simulink model "humanSubject07_48dof_test"  (R2022a)
settings: Solver=VariableStepAuto  StartTime=0.0  StopTime=4.5  RelTol=1e-3
values from neighbouring files (symbols this model uses):
  m = size(marker.links, 1)    [master_thesis_script.m]    (also in trial.m)
  marker = msg.ChildFrameId(14)    [callback_class.m]
  noise =     [noise_S1_F1_H2.mat]    (also in show_Results.m = noise.noise)
  s = s + 1    (= 2)    [Phi_J_generation.m]    (also in master_thesis_script.m; trial.m)
undefined symbols (not defined in the file or in its folder): arm, LS, X, Y, Z
libraries: nesl_utility x105, sm_lib x84
(part 2 of 3)

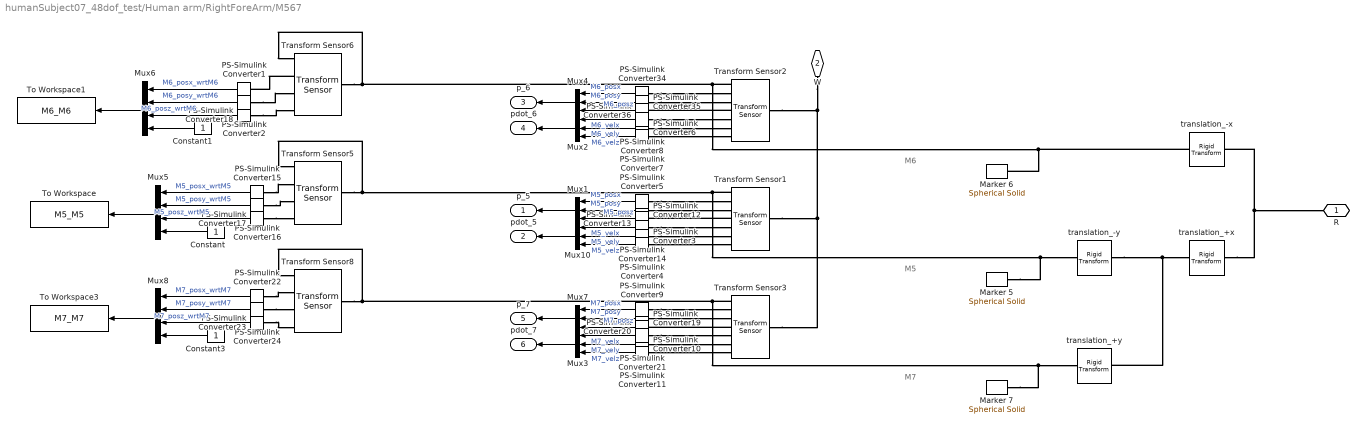
== system humanSubject07_48dof_test/Human arm/RightForeArm/M567 ==
  note: M6
  note: M5
  note: M7
  Constant : Constant
  Constant1 : Constant
  Constant3 : Constant
  Marker 5 : sm_lib/Body Elements/Spherical Solid  GraphicAmbientColor=[0.15 0.15 0.15 1.0]  BasedOnType=Density  CenterOfMass=[0 0 0]  CenterOfMassUnits=m  GraphicDiffuseColor=[1.0 0.2 0.2]  Density=1000  DensityUnits=kg/m^3  DoExposeReferenceFrame=on  GraphicEmissiveColor=[0.0 0.0 0.0 1.0]  ExportEntireGeometry=off  SerializedExposedGeometries=<ExposedGeometries/>  SerializedFrames=<Frames/>  MarkerShape=Sphere  MarkerSize=10  GraphicType=FromGeometry  InertiaType=CalculateFromGeometry  Mass=1  MassUnits=kg  MomentsOfInertia=[1 1 1]  MomentsOfInertiaUnits=kg*m^2  GraphicOpacity=1.0  ProductsOfInertia=[0 0 0]  ProductsOfInertiaUnits=kg*m^2  GraphicShininess=75  GraphicSpecularColor=[0.5 0.5 0.5 1.0]  SphereRadius=arm.markers.radius  SphereRadiusUnits=m  GraphicVisPropType=SimpleVisualProperties
  Marker 6 : sm_lib/Body Elements/Spherical Solid  GraphicAmbientColor=[0.15 0.15 0.15 1.0]  BasedOnType=Density  CenterOfMass=[0 0 0]  CenterOfMassUnits=m  GraphicDiffuseColor=[1.0 0.2 0.2]  Density=1000  DensityUnits=kg/m^3  DoExposeReferenceFrame=on  GraphicEmissiveColor=[0.0 0.0 0.0 1.0]  ExportEntireGeometry=off  SerializedExposedGeometries=<ExposedGeometries/>  SerializedFrames=<Frames/>  MarkerShape=Sphere  MarkerSize=10  GraphicType=FromGeometry  InertiaType=CalculateFromGeometry  Mass=1  MassUnits=kg  MomentsOfInertia=[1 1 1]  MomentsOfInertiaUnits=kg*m^2  GraphicOpacity=1.0  ProductsOfInertia=[0 0 0]  ProductsOfInertiaUnits=kg*m^2  GraphicShininess=75  GraphicSpecularColor=[0.5 0.5 0.5 1.0]  SphereRadius=arm.markers.radius  SphereRadiusUnits=m  GraphicVisPropType=SimpleVisualProperties
  Marker 7 : sm_lib/Body Elements/Spherical Solid  GraphicAmbientColor=[0.15 0.15 0.15 1.0]  BasedOnType=Density  CenterOfMass=[0 0 0]  CenterOfMassUnits=m  GraphicDiffuseColor=[1.0 0.2 0.2]  Density=1000  DensityUnits=kg/m^3  DoExposeReferenceFrame=on  GraphicEmissiveColor=[0.0 0.0 0.0 1.0]  ExportEntireGeometry=off  SerializedExposedGeometries=<ExposedGeometries/>  SerializedFrames=<Frames/>  MarkerShape=Sphere  MarkerSize=10  GraphicType=FromGeometry  InertiaType=CalculateFromGeometry  Mass=1  MassUnits=kg  MomentsOfInertia=[1 1 1]  MomentsOfInertiaUnits=kg*m^2  GraphicOpacity=1.0  ProductsOfInertia=[0 0 0]  ProductsOfInertiaUnits=kg*m^2  GraphicShininess=75  GraphicSpecularColor=[0.5 0.5 0.5 1.0]  SphereRadius=arm.markers.radius  SphereRadiusUnits=m  GraphicVisPropType=SimpleVisualProperties
  Mux{1..4,7,10} (6 alike) : Mux  Inputs=3
  Mux5 : Mux
  Mux6 : Mux
  Mux8 : Mux
  PS-Simulink Converter{1..24,34..36} (27 alike) : nesl_utility/PS-Simulink Converter  PhysicalDomain=network_engine_domain  SubClassName=ps_output  LeftPortType=input  RightPortType=output  PseudoPeriodic=off  Frequencies=[]  VectorFormat=inherit  Unit=inherit  AffineConversion=off
      settings: SourceProductBaseCode=SS,PW,VE
  To Workspace : ToWorkspace  VariableName=M5_M5  SaveFormat=Structure With Time  SampleTime=-1
  To Workspace1 : ToWorkspace  VariableName=M6_M6  SaveFormat=Structure With Time  SampleTime=-1
  To Workspace3 : ToWorkspace  VariableName=M7_M7  SaveFormat=Structure With Time  SampleTime=-1
  Transform Sensor1 : sm_lib/Frames and Transforms/Transform Sensor  MeasurementFrame=World  SenseAngle=off  SenseAxis=off  SenseAngle1=off  SenseAngle2=off  SenseAngle3=off  SenseQ=off  SenseR=off  SenseOmegaX=off  SenseOmegaY=off  SenseOmegaZ=off  SenseOmega1=off  SenseOmega2=off  SenseOmega3=off  SenseQDot=off  SenseRDot=off  SenseAlphaX=off  SenseAlphaY=off  SenseAlphaZ=off  SenseAlpha1=off  SenseAlpha2=off  SenseAlpha3=off  SenseQDDot=off  SenseRDDot=off  SenseX=on  SenseY=on  SenseZ=on  SenseRad=off  SenseAzim=off  SenseDist=off  SenseInc=off  SenseXDot=on  SenseYDot=on  SenseZDot=on  SenseRadDot=off  SenseAzimDot=off  SenseDistDot=off  SenseIncDot=off  SenseXDDot=off  SenseYDDot=off  SenseZDDot=off  SenseRadDDot=off  SenseAzimDDot=off  SenseDistDDot=off  SenseIncDDot=off
  Transform Sensor2 : sm_lib/Frames and Transforms/Transform Sensor  MeasurementFrame=World  SenseAngle=off  SenseAxis=off  SenseAngle1=off  SenseAngle2=off  SenseAngle3=off  SenseQ=off  SenseR=off  SenseOmegaX=off  SenseOmegaY=off  SenseOmegaZ=off  SenseOmega1=off  SenseOmega2=off  SenseOmega3=off  SenseQDot=off  SenseRDot=off  SenseAlphaX=off  SenseAlphaY=off  SenseAlphaZ=off  SenseAlpha1=off  SenseAlpha2=off  SenseAlpha3=off  SenseQDDot=off  SenseRDDot=off  SenseX=on  SenseY=on  SenseZ=on  SenseRad=off  SenseAzim=off  SenseDist=off  SenseInc=off  SenseXDot=on  SenseYDot=on  SenseZDot=on  SenseRadDot=off  SenseAzimDot=off  SenseDistDot=off  SenseIncDot=off  SenseXDDot=off  SenseYDDot=off  SenseZDDot=off  SenseRadDDot=off  SenseAzimDDot=off  SenseDistDDot=off  SenseIncDDot=off
  Transform Sensor3 : sm_lib/Frames and Transforms/Transform Sensor  MeasurementFrame=World  SenseAngle=off  SenseAxis=off  SenseAngle1=off  SenseAngle2=off  SenseAngle3=off  SenseQ=off  SenseR=off  SenseOmegaX=off  SenseOmegaY=off  SenseOmegaZ=off  SenseOmega1=off  SenseOmega2=off  SenseOmega3=off  SenseQDot=off  SenseRDot=off  SenseAlphaX=off  SenseAlphaY=off  SenseAlphaZ=off  SenseAlpha1=off  SenseAlpha2=off  SenseAlpha3=off  SenseQDDot=off  SenseRDDot=off  SenseX=on  SenseY=on  SenseZ=on  SenseRad=off  SenseAzim=off  SenseDist=off  SenseInc=off  SenseXDot=on  SenseYDot=on  SenseZDot=on  SenseRadDot=off  SenseAzimDot=off  SenseDistDot=off  SenseIncDot=off  SenseXDDot=off  SenseYDDot=off  SenseZDDot=off  SenseRadDDot=off  SenseAzimDDot=off  SenseDistDDot=off  SenseIncDDot=off
  Transform Sensor5 : sm_lib/Frames and Transforms/Transform Sensor  MeasurementFrame=World  SenseAngle=off  SenseAxis=off  SenseAngle1=off  SenseAngle2=off  SenseAngle3=off  SenseQ=off  SenseR=off  SenseOmegaX=off  SenseOmegaY=off  SenseOmegaZ=off  SenseOmega1=off  SenseOmega2=off  SenseOmega3=off  SenseQDot=off  SenseRDot=off  SenseAlphaX=off  SenseAlphaY=off  SenseAlphaZ=off  SenseAlpha1=off  SenseAlpha2=off  SenseAlpha3=off  SenseQDDot=off  SenseRDDot=off  SenseX=on  SenseY=on  SenseZ=on  SenseRad=off  SenseAzim=off  SenseDist=off  SenseInc=off  SenseXDot=off  SenseYDot=off  SenseZDot=off  SenseRadDot=off  SenseAzimDot=off  SenseDistDot=off  SenseIncDot=off  SenseXDDot=off  SenseYDDot=off  SenseZDDot=off  SenseRadDDot=off  SenseAzimDDot=off  SenseDistDDot=off  SenseIncDDot=off
  Transform Sensor6 : sm_lib/Frames and Transforms/Transform Sensor  MeasurementFrame=World  SenseAngle=off  SenseAxis=off  SenseAngle1=off  SenseAngle2=off  SenseAngle3=off  SenseQ=off  SenseR=off  SenseOmegaX=off  SenseOmegaY=off  SenseOmegaZ=off  SenseOmega1=off  SenseOmega2=off  SenseOmega3=off  SenseQDot=off  SenseRDot=off  SenseAlphaX=off  SenseAlphaY=off  SenseAlphaZ=off  SenseAlpha1=off  SenseAlpha2=off  SenseAlpha3=off  SenseQDDot=off  SenseRDDot=off  SenseX=on  SenseY=on  SenseZ=on  SenseRad=off  SenseAzim=off  SenseDist=off  SenseInc=off  SenseXDot=off  SenseYDot=off  SenseZDot=off  SenseRadDot=off  SenseAzimDot=off  SenseDistDot=off  SenseIncDot=off  SenseXDDot=off  SenseYDDot=off  SenseZDDot=off  SenseRadDDot=off  SenseAzimDDot=off  SenseDistDDot=off  SenseIncDDot=off
  Transform Sensor8 : sm_lib/Frames and Transforms/Transform Sensor  MeasurementFrame=World  SenseAngle=off  SenseAxis=off  SenseAngle1=off  SenseAngle2=off  SenseAngle3=off  SenseQ=off  SenseR=off  SenseOmegaX=off  SenseOmegaY=off  SenseOmegaZ=off  SenseOmega1=off  SenseOmega2=off  SenseOmega3=off  SenseQDot=off  SenseRDot=off  SenseAlphaX=off  SenseAlphaY=off  SenseAlphaZ=off  SenseAlpha1=off  SenseAlpha2=off  SenseAlpha3=off  SenseQDDot=off  SenseRDDot=off  SenseX=on  SenseY=on  SenseZ=on  SenseRad=off  SenseAzim=off  SenseDist=off  SenseInc=off  SenseXDot=off  SenseYDot=off  SenseZDot=off  SenseRadDot=off  SenseAzimDot=off  SenseDistDot=off  SenseIncDot=off  SenseXDDot=off  SenseYDDot=off  SenseZDDot=off  SenseRadDDot=off  SenseAzimDDot=off  SenseDistDDot=off  SenseIncDDot=off
  translation_+x : sm_lib/Frames and Transforms/Rigid Transform  TranslationMethod=Cartesian  TranslationStandardOffset=0  TranslationLengthUnit=m  TranslationStandardAxis=+Z  TranslationCartesianOffset=[arm.forearm.radius+arm.markers.radius 0 0]  TranslationROffset=0  TranslationROffsetUnits=m  TranslationZOffset=0  TranslationZOffsetUnits=m  TranslationThetaOffset=0  TranslationThetaOffsetUnits=deg  RotationMethod=None  RotationAngleUnits=rad  RotationStandardAxis=+Z  RotationAngle=pi/2  RotationArbitraryAxis=[1 0 0]  FollAlignAxisA=+X  BaseAlignAxisA=+Y  FollAlignAxisB=+Y  BaseAlignAxisB=+Z  RotationSequenceAxes=BaseAxes  RotationSequence=XYZ  RotationSequenceAngles=[pi/2, 0, 0]  RotationSequenceAnglesUnits=rad  RotationMatrix=[1 0 0; 0 1 0; 0 0 1]
  translation_+y : sm_lib/Frames and Transforms/Rigid Transform  TranslationMethod=Cartesian  TranslationStandardOffset=0  TranslationLengthUnit=m  TranslationStandardAxis=+Z  TranslationCartesianOffset=[0 arm.forearm.length/4 0]  TranslationROffset=0  TranslationROffsetUnits=m  TranslationZOffset=0  TranslationZOffsetUnits=m  TranslationThetaOffset=0  TranslationThetaOffsetUnits=deg  RotationMethod=None  RotationAngleUnits=rad  RotationStandardAxis=+Z  RotationAngle=pi/2  RotationArbitraryAxis=[1 0 0]  FollAlignAxisA=+X  BaseAlignAxisA=+Y  FollAlignAxisB=+Y  BaseAlignAxisB=+Z  RotationSequenceAxes=BaseAxes  RotationSequence=XYZ  RotationSequenceAngles=[pi/2, 0, 0]  RotationSequenceAnglesUnits=rad  RotationMatrix=[1 0 0; 0 1 0; 0 0 1]
  translation_-x : sm_lib/Frames and Transforms/Rigid Transform  TranslationMethod=Cartesian  TranslationStandardOffset=0  TranslationLengthUnit=m  TranslationStandardAxis=+Z  TranslationCartesianOffset=[-arm.forearm.radius-arm.markers.radius 0 0]  TranslationROffset=0  TranslationROffsetUnits=m  TranslationZOffset=0  TranslationZOffsetUnits=m  TranslationThetaOffset=0  TranslationThetaOffsetUnits=deg  RotationMethod=None  RotationAngleUnits=rad  RotationStandardAxis=+Z  RotationAngle=pi/2  RotationArbitraryAxis=[1 0 0]  FollAlignAxisA=+X  BaseAlignAxisA=+Y  FollAlignAxisB=+Y  BaseAlignAxisB=+Z  RotationSequenceAxes=BaseAxes  RotationSequence=XYZ  RotationSequenceAngles=[pi/2, 0, 0]  RotationSequenceAnglesUnits=rad  RotationMatrix=[1 0 0; 0 1 0; 0 0 1]
  translation_-y : sm_lib/Frames and Transforms/Rigid Transform  TranslationMethod=Cartesian  TranslationStandardOffset=0  TranslationLengthUnit=m  TranslationStandardAxis=+Z  TranslationCartesianOffset=[0 -arm.forearm.length/4 0]  TranslationROffset=0  TranslationROffsetUnits=m  TranslationZOffset=0  TranslationZOffsetUnits=m  TranslationThetaOffset=0  TranslationThetaOffsetUnits=deg  RotationMethod=None  RotationAngleUnits=rad  RotationStandardAxis=+Z  RotationAngle=pi/2  RotationArbitraryAxis=[1 0 0]  FollAlignAxisA=+X  BaseAlignAxisA=+Y  FollAlignAxisB=+Y  BaseAlignAxisB=+Z  RotationSequenceAxes=BaseAxes  RotationSequence=XYZ  RotationSequenceAngles=[pi/2, 0, 0]  RotationSequenceAnglesUnits=rad  RotationMatrix=[1 0 0; 0 1 0; 0 0 1]
  R : PMIOPort  Side=Left
  W : PMIOPort  Port=2  Side=Left
  p_5 : Outport
  pdot_5 : Outport  Port=2
  p_6 : Outport  Port=3
  pdot_6 : Outport  Port=4
  p_7 : Outport  Port=5
  pdot_7 : Outport  Port=6
  wires:
  Mux5/1 -> To Workspace/1
  PS-Simulink Converter17/1 -> Mux5/3  "M5_posz_wrtM5"
  PS-Simulink Converter15/1 -> Mux5/1  "M5_posx_wrtM5"
  PS-Simulink Converter16/1 -> Mux5/2  "M5_posy_wrtM5"
  Constant/1 -> Mux5/4
  Mux6/1 -> To Workspace1/1
  PS-Simulink Converter1/1 -> Mux6/1  "M6_posx_wrtM6"
  PS-Simulink Converter2/1 -> Mux6/2  "M6_posy_wrtM6"
  Constant1/1 -> Mux6/4
  PS-Simulink Converter18/1 -> Mux6/3  "M6_posz_wrtM6"
  Constant3/1 -> Mux8/4
  PS-Simulink Converter22/1 -> Mux8/1  "M7_posx_wrtM7"
  PS-Simulink Converter24/1 -> Mux8/2  "M7_posy_wrtM7"
  Mux8/1 -> To Workspace3/1
  PS-Simulink Converter23/1 -> Mux8/3  "M7_posz_wrtM7"
  PS-Simulink Converter35/1 -> Mux4/2  "M6_posy"
  PS-Simulink Converter34/1 -> Mux4/1  "M6_posx"
  PS-Simulink Converter8/1 -> Mux2/1  "M6_velx"
  PS-Simulink Converter6/1 -> Mux2/2  "M6_vely"
  PS-Simulink Converter36/1 -> Mux4/3  "M6_posz"
  PS-Simulink Converter7/1 -> Mux2/3  "M6_velz"
  PS-Simulink Converter12/1 -> Mux1/2  "M5_posy"
  PS-Simulink Converter5/1 -> Mux1/1  "M5_posx"
  PS-Simulink Converter14/1 -> Mux10/1  "M5_velx"
  PS-Simulink Converter3/1 -> Mux10/2  "M5_vely"
  PS-Simulink Converter13/1 -> Mux1/3  "M5_posz"
  PS-Simulink Converter4/1 -> Mux10/3  "M5_velz"
  PS-Simulink Converter19/1 -> Mux7/2  "M7_posy"
  PS-Simulink Converter9/1 -> Mux7/1  "M7_posx"
  PS-Simulink Converter21/1 -> Mux3/1  "M7_velx"
  PS-Simulink Converter10/1 -> Mux3/2  "M7_vely"
  PS-Simulink Converter20/1 -> Mux7/3  "M7_posz"
  PS-Simulink Converter11/1 -> Mux3/3  "M7_velz"
  Mux1/1 -> p_5/1
  Mux10/1 -> pdot_5/1
  Mux4/1 -> p_6/1
  Mux2/1 -> pdot_6/1
  Mux7/1 -> p_7/1
  Mux3/1 -> pdot_7/1
  connections:
  translation_+x/LConn1 -- translation_-x/LConn1 -- R/RConn1
  translation_-y/LConn1 -- translation_+y/LConn1 -- translation_+x/RConn1
  Transform Sensor2/RConn1 -- Transform Sensor6/RConn1 -- Transform Sensor6/LConn1 -- Marker 6/RConn1 -- translation_-x/RConn1
  W/RConn1 -- Transform Sensor3/LConn1 -- Transform Sensor1/LConn1 -- Transform Sensor2/LConn1
  PS-Simulink Converter16/LConn1 -- Transform Sensor5/RConn3
  PS-Simulink Converter17/LConn1 -- Transform Sensor5/RConn4
  PS-Simulink Converter15/LConn1 -- Transform Sensor5/RConn2
  Transform Sensor6/RConn2 -- PS-Simulink Converter1/LConn1
  PS-Simulink Converter18/LConn1 -- Transform Sensor6/RConn4
  PS-Simulink Converter2/LConn1 -- Transform Sensor6/RConn3
  PS-Simulink Converter24/LConn1 -- Transform Sensor8/RConn3
  PS-Simulink Converter23/LConn1 -- Transform Sensor8/RConn4
  PS-Simulink Converter22/LConn1 -- Transform Sensor8/RConn2
  PS-Simulink Converter35/LConn1 -- Transform Sensor2/RConn3
  PS-Simulink Converter34/LConn1 -- Transform Sensor2/RConn2
  PS-Simulink Converter8/LConn1 -- Transform Sensor2/RConn5
  PS-Simulink Converter6/LConn1 -- Transform Sensor2/RConn6
  PS-Simulink Converter7/LConn1 -- Transform Sensor2/RConn7
  Transform Sensor2/RConn4 -- PS-Simulink Converter36/LConn1
  Transform Sensor5/LConn1 -- Transform Sensor5/RConn1 -- translation_-y/RConn1 -- Marker 5/RConn1 -- Transform Sensor1/RConn1
  PS-Simulink Converter12/LConn1 -- Transform Sensor1/RConn3
  PS-Simulink Converter5/LConn1 -- Transform Sensor1/RConn2
  PS-Simulink Converter14/LConn1 -- Transform Sensor1/RConn5
  PS-Simulink Converter3/LConn1 -- Transform Sensor1/RConn6
  PS-Simulink Converter4/LConn1 -- Transform Sensor1/RConn7
  Transform Sensor1/RConn4 -- PS-Simulink Converter13/LConn1
  Transform Sensor3/RConn1 -- Transform Sensor8/RConn1 -- Transform Sensor8/LConn1 -- translation_+y/RConn1 -- Marker 7/RConn1
  PS-Simulink Converter19/LConn1 -- Transform Sensor3/RConn3
  PS-Simulink Converter9/LConn1 -- Transform Sensor3/RConn2
  PS-Simulink Converter21/LConn1 -- Transform Sensor3/RConn5
  PS-Simulink Converter10/LConn1 -- Transform Sensor3/RConn6
  PS-Simulink Converter11/LConn1 -- Transform Sensor3/RConn7
  Transform Sensor3/RConn4 -- PS-Simulink Converter20/LConn1

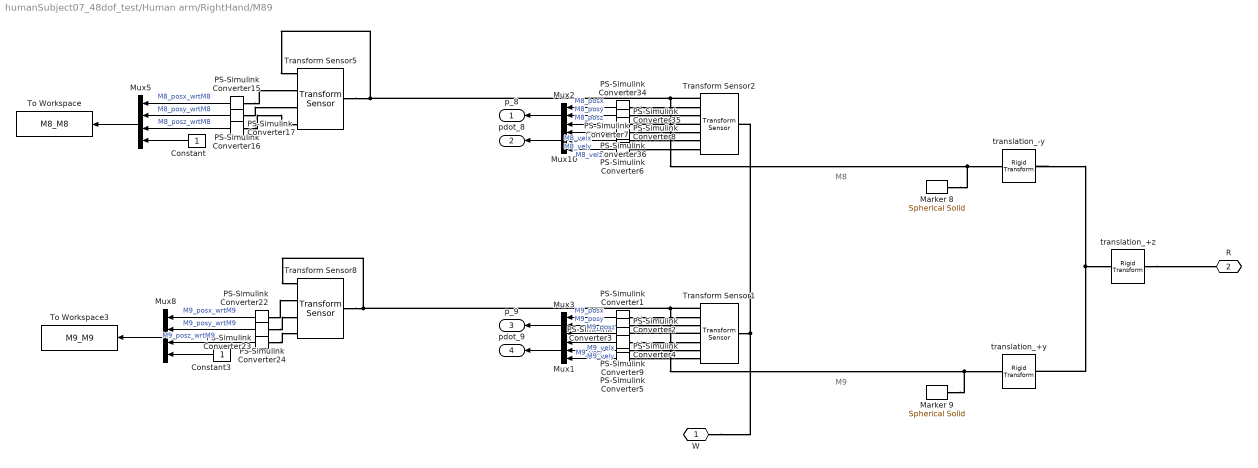
== system humanSubject07_48dof_test/Human arm/RightHand/M89 ==
  note: M8
  note: M9
  Constant : Constant
  Constant3 : Constant
  Marker 8 : sm_lib/Body Elements/Spherical Solid  GraphicAmbientColor=[0.15 0.15 0.15 1.0]  BasedOnType=Density  CenterOfMass=[0 0 0]  CenterOfMassUnits=m  GraphicDiffuseColor=[1.0 0.2 0.2]  Density=1000  DensityUnits=kg/m^3  DoExposeReferenceFrame=on  GraphicEmissiveColor=[0.0 0.0 0.0 1.0]  ExportEntireGeometry=off  SerializedExposedGeometries=<ExposedGeometries/>  SerializedFrames=<Frames/>  MarkerShape=Sphere  MarkerSize=10  GraphicType=FromGeometry  InertiaType=CalculateFromGeometry  Mass=1  MassUnits=kg  MomentsOfInertia=[1 1 1]  MomentsOfInertiaUnits=kg*m^2  GraphicOpacity=1.0  ProductsOfInertia=[0 0 0]  ProductsOfInertiaUnits=kg*m^2  GraphicShininess=75  GraphicSpecularColor=[0.5 0.5 0.5 1.0]  SphereRadius=arm.markers.radius  SphereRadiusUnits=m  GraphicVisPropType=SimpleVisualProperties
  Marker 9 : sm_lib/Body Elements/Spherical Solid  GraphicAmbientColor=[0.15 0.15 0.15 1.0]  BasedOnType=Density  CenterOfMass=[0 0 0]  CenterOfMassUnits=m  GraphicDiffuseColor=[1.0 0.2 0.2]  Density=1000  DensityUnits=kg/m^3  DoExposeReferenceFrame=on  GraphicEmissiveColor=[0.0 0.0 0.0 1.0]  ExportEntireGeometry=off  SerializedExposedGeometries=<ExposedGeometries/>  SerializedFrames=<Frames/>  MarkerShape=Sphere  MarkerSize=10  GraphicType=FromGeometry  InertiaType=CalculateFromGeometry  Mass=1  MassUnits=kg  MomentsOfInertia=[1 1 1]  MomentsOfInertiaUnits=kg*m^2  GraphicOpacity=1.0  ProductsOfInertia=[0 0 0]  ProductsOfInertiaUnits=kg*m^2  GraphicShininess=75  GraphicSpecularColor=[0.5 0.5 0.5 1.0]  SphereRadius=arm.markers.radius  SphereRadiusUnits=m  GraphicVisPropType=SimpleVisualProperties
  Mux{1..3,10} (4 alike) : Mux  Inputs=3
  Mux5 : Mux
  Mux8 : Mux
  PS-Simulink Converter{1..9,15..17,22..24,34..36} (18 alike) : nesl_utility/PS-Simulink Converter  PhysicalDomain=network_engine_domain  SubClassName=ps_output  LeftPortType=input  RightPortType=output  PseudoPeriodic=off  Frequencies=[]  VectorFormat=inherit  Unit=inherit  AffineConversion=off
      settings: SourceProductBaseCode=SS,PW,VE
  To Workspace : ToWorkspace  VariableName=M8_M8  SaveFormat=Structure With Time  SampleTime=-1
  To Workspace3 : ToWorkspace  VariableName=M9_M9  SaveFormat=Structure With Time  SampleTime=-1
  Transform Sensor1 : sm_lib/Frames and Transforms/Transform Sensor  MeasurementFrame=World  SenseAngle=off  SenseAxis=off  SenseAngle1=off  SenseAngle2=off  SenseAngle3=off  SenseQ=off  SenseR=off  SenseOmegaX=off  SenseOmegaY=off  SenseOmegaZ=off  SenseOmega1=off  SenseOmega2=off  SenseOmega3=off  SenseQDot=off  SenseRDot=off  SenseAlphaX=off  SenseAlphaY=off  SenseAlphaZ=off  SenseAlpha1=off  SenseAlpha2=off  SenseAlpha3=off  SenseQDDot=off  SenseRDDot=off  SenseX=on  SenseY=on  SenseZ=on  SenseRad=off  SenseAzim=off  SenseDist=off  SenseInc=off  SenseXDot=on  SenseYDot=on  SenseZDot=on  SenseRadDot=off  SenseAzimDot=off  SenseDistDot=off  SenseIncDot=off  SenseXDDot=off  SenseYDDot=off  SenseZDDot=off  SenseRadDDot=off  SenseAzimDDot=off  SenseDistDDot=off  SenseIncDDot=off
  Transform Sensor2 : sm_lib/Frames and Transforms/Transform Sensor  MeasurementFrame=World  SenseAngle=off  SenseAxis=off  SenseAngle1=off  SenseAngle2=off  SenseAngle3=off  SenseQ=off  SenseR=off  SenseOmegaX=off  SenseOmegaY=off  SenseOmegaZ=off  SenseOmega1=off  SenseOmega2=off  SenseOmega3=off  SenseQDot=off  SenseRDot=off  SenseAlphaX=off  SenseAlphaY=off  SenseAlphaZ=off  SenseAlpha1=off  SenseAlpha2=off  SenseAlpha3=off  SenseQDDot=off  SenseRDDot=off  SenseX=on  SenseY=on  SenseZ=on  SenseRad=off  SenseAzim=off  SenseDist=off  SenseInc=off  SenseXDot=on  SenseYDot=on  SenseZDot=on  SenseRadDot=off  SenseAzimDot=off  SenseDistDot=off  SenseIncDot=off  SenseXDDot=off  SenseYDDot=off  SenseZDDot=off  SenseRadDDot=off  SenseAzimDDot=off  SenseDistDDot=off  SenseIncDDot=off
  Transform Sensor5 : sm_lib/Frames and Transforms/Transform Sensor  MeasurementFrame=World  SenseAngle=off  SenseAxis=off  SenseAngle1=off  SenseAngle2=off  SenseAngle3=off  SenseQ=off  SenseR=off  SenseOmegaX=off  SenseOmegaY=off  SenseOmegaZ=off  SenseOmega1=off  SenseOmega2=off  SenseOmega3=off  SenseQDot=off  SenseRDot=off  SenseAlphaX=off  SenseAlphaY=off  SenseAlphaZ=off  SenseAlpha1=off  SenseAlpha2=off  SenseAlpha3=off  SenseQDDot=off  SenseRDDot=off  SenseX=on  SenseY=on  SenseZ=on  SenseRad=off  SenseAzim=off  SenseDist=off  SenseInc=off  SenseXDot=off  SenseYDot=off  SenseZDot=off  SenseRadDot=off  SenseAzimDot=off  SenseDistDot=off  SenseIncDot=off  SenseXDDot=off  SenseYDDot=off  SenseZDDot=off  SenseRadDDot=off  SenseAzimDDot=off  SenseDistDDot=off  SenseIncDDot=off
  Transform Sensor8 : sm_lib/Frames and Transforms/Transform Sensor  MeasurementFrame=World  SenseAngle=off  SenseAxis=off  SenseAngle1=off  SenseAngle2=off  SenseAngle3=off  SenseQ=off  SenseR=off  SenseOmegaX=off  SenseOmegaY=off  SenseOmegaZ=off  SenseOmega1=off  SenseOmega2=off  SenseOmega3=off  SenseQDot=off  SenseRDot=off  SenseAlphaX=off  SenseAlphaY=off  SenseAlphaZ=off  SenseAlpha1=off  SenseAlpha2=off  SenseAlpha3=off  SenseQDDot=off  SenseRDDot=off  SenseX=on  SenseY=on  SenseZ=on  SenseRad=off  SenseAzim=off  SenseDist=off  SenseInc=off  SenseXDot=off  SenseYDot=off  SenseZDot=off  SenseRadDot=off  SenseAzimDot=off  SenseDistDot=off  SenseIncDot=off  SenseXDDot=off  SenseYDDot=off  SenseZDDot=off  SenseRadDDot=off  SenseAzimDDot=off  SenseDistDDot=off  SenseIncDDot=off
  translation_+y : sm_lib/Frames and Transforms/Rigid Transform  TranslationMethod=Cartesian  TranslationStandardOffset=0  TranslationLengthUnit=m  TranslationStandardAxis=+Z  TranslationCartesianOffset=[0 arm.hand.dimensions(2)/4 0]  TranslationROffset=0  TranslationROffsetUnits=m  TranslationZOffset=0  TranslationZOffsetUnits=m  TranslationThetaOffset=0  TranslationThetaOffsetUnits=deg  RotationMethod=None  RotationAngleUnits=rad  RotationStandardAxis=+Z  RotationAngle=pi/2  RotationArbitraryAxis=[1 0 0]  FollAlignAxisA=+X  BaseAlignAxisA=+Y  FollAlignAxisB=+Y  BaseAlignAxisB=+Z  RotationSequenceAxes=BaseAxes  RotationSequence=XYZ  RotationSequenceAngles=[pi/2, 0, 0]  RotationSequenceAnglesUnits=rad  RotationMatrix=[1 0 0; 0 1 0; 0 0 1]
  translation_+z : sm_lib/Frames and Transforms/Rigid Transform  TranslationMethod=Cartesian  TranslationStandardOffset=0  TranslationLengthUnit=m  TranslationStandardAxis=+Z  TranslationCartesianOffset=[0 0 arm.hand.dimensions(3)/2+arm.markers.radius]  TranslationROffset=0  TranslationROffsetUnits=m  TranslationZOffset=0  TranslationZOffsetUnits=m  TranslationThetaOffset=0  TranslationThetaOffsetUnits=deg  RotationMethod=None  RotationAngleUnits=rad  RotationStandardAxis=+Z  RotationAngle=pi/2  RotationArbitraryAxis=[1 0 0]  FollAlignAxisA=+X  BaseAlignAxisA=+Y  FollAlignAxisB=+Y  BaseAlignAxisB=+Z  RotationSequenceAxes=BaseAxes  RotationSequence=XYZ  RotationSequenceAngles=[pi/2, 0, 0]  RotationSequenceAnglesUnits=rad  RotationMatrix=[1 0 0; 0 1 0; 0 0 1]
  translation_-y : sm_lib/Frames and Transforms/Rigid Transform  TranslationMethod=Cartesian  TranslationStandardOffset=0  TranslationLengthUnit=m  TranslationStandardAxis=+Z  TranslationCartesianOffset=[0 -arm.hand.dimensions(2)/4 0]  TranslationROffset=0  TranslationROffsetUnits=m  TranslationZOffset=0  TranslationZOffsetUnits=m  TranslationThetaOffset=0  TranslationThetaOffsetUnits=deg  RotationMethod=None  RotationAngleUnits=rad  RotationStandardAxis=+Z  RotationAngle=pi/2  RotationArbitraryAxis=[1 0 0]  FollAlignAxisA=+X  BaseAlignAxisA=+Y  FollAlignAxisB=+Y  BaseAlignAxisB=+Z  RotationSequenceAxes=BaseAxes  RotationSequence=XYZ  RotationSequenceAngles=[pi/2, 0, 0]  RotationSequenceAnglesUnits=rad  RotationMatrix=[1 0 0; 0 1 0; 0 0 1]
  W : PMIOPort  Side=Left
  R : PMIOPort  Port=2  Side=Left
  p_8 : Outport
  pdot_8 : Outport  Port=2
  p_9 : Outport  Port=3
  pdot_9 : Outport  Port=4
  wires:
  Mux5/1 -> To Workspace/1
  PS-Simulink Converter17/1 -> Mux5/3  "M8_posz_wrtM8"
  PS-Simulink Converter15/1 -> Mux5/1  "M8_posx_wrtM8"
  PS-Simulink Converter16/1 -> Mux5/2  "M8_posy_wrtM8"
  Constant/1 -> Mux5/4
  Constant3/1 -> Mux8/4
  PS-Simulink Converter22/1 -> Mux8/1  "M9_posx_wrtM9"
  PS-Simulink Converter24/1 -> Mux8/2  "M9_posy_wrtM9"
  Mux8/1 -> To Workspace3/1
  PS-Simulink Converter23/1 -> Mux8/3  "M9_posz_wrtM9"
  PS-Simulink Converter8/1 -> Mux10/1  "M8_velx"
  PS-Simulink Converter6/1 -> Mux10/2  "M8_vely"
  PS-Simulink Converter36/1 -> Mux2/3  "M8_posz"
  PS-Simulink Converter35/1 -> Mux2/2  "M8_posy"
  PS-Simulink Converter7/1 -> Mux10/3  "M8_velz"
  PS-Simulink Converter34/1 -> Mux2/1  "M8_posx"
  PS-Simulink Converter5/1 -> Mux1/3  "M9_velz"
  PS-Simulink Converter1/1 -> Mux3/1  "M9_posx"
  PS-Simulink Converter9/1 -> Mux1/1  "M9_velx"
  PS-Simulink Converter4/1 -> Mux1/2  "M9_vely"
  PS-Simulink Converter3/1 -> Mux3/3  "M9_posz"
  PS-Simulink Converter2/1 -> Mux3/2  "M9_posy"
  Mux2/1 -> p_8/1
  Mux10/1 -> pdot_8/1
  Mux3/1 -> p_9/1
  Mux1/1 -> pdot_9/1
  connections:
  translation_-y/LConn1 -- translation_+y/LConn1 -- translation_+z/RConn1
  Transform Sensor1/RConn1 -- Transform Sensor8/RConn1 -- Transform Sensor8/LConn1 -- translation_+y/RConn1 -- Marker 9/RConn1
  W/RConn1 -- Transform Sensor1/LConn1 -- Transform Sensor2/LConn1
  PS-Simulink Converter16/LConn1 -- Transform Sensor5/RConn3
  PS-Simulink Converter17/LConn1 -- Transform Sensor5/RConn4
  PS-Simulink Converter15/LConn1 -- Transform Sensor5/RConn2
  PS-Simulink Converter24/LConn1 -- Transform Sensor8/RConn3
  PS-Simulink Converter23/LConn1 -- Transform Sensor8/RConn4
  PS-Simulink Converter22/LConn1 -- Transform Sensor8/RConn2
  translation_+z/LConn1 -- R/RConn1
  Transform Sensor2/RConn1 -- translation_-y/RConn1 -- Marker 8/RConn1 -- Transform Sensor5/RConn1 -- Transform Sensor5/LConn1
  PS-Simulink Converter8/LConn1 -- Transform Sensor2/RConn5
  Transform Sensor2/RConn4 -- PS-Simulink Converter36/LConn1
  PS-Simulink Converter35/LConn1 -- Transform Sensor2/RConn3
  PS-Simulink Converter34/LConn1 -- Transform Sensor2/RConn2
  PS-Simulink Converter6/LConn1 -- Transform Sensor2/RConn6
  PS-Simulink Converter7/LConn1 -- Transform Sensor2/RConn7
  PS-Simulink Converter5/LConn1 -- Transform Sensor1/RConn7
  PS-Simulink Converter9/LConn1 -- Transform Sensor1/RConn5
  PS-Simulink Converter1/LConn1 -- Transform Sensor1/RConn2
  Transform Sensor1/RConn4 -- PS-Simulink Converter3/LConn1
  PS-Simulink Converter2/LConn1 -- Transform Sensor1/RConn3
  PS-Simulink Converter4/LConn1 -- Transform Sensor1/RConn6

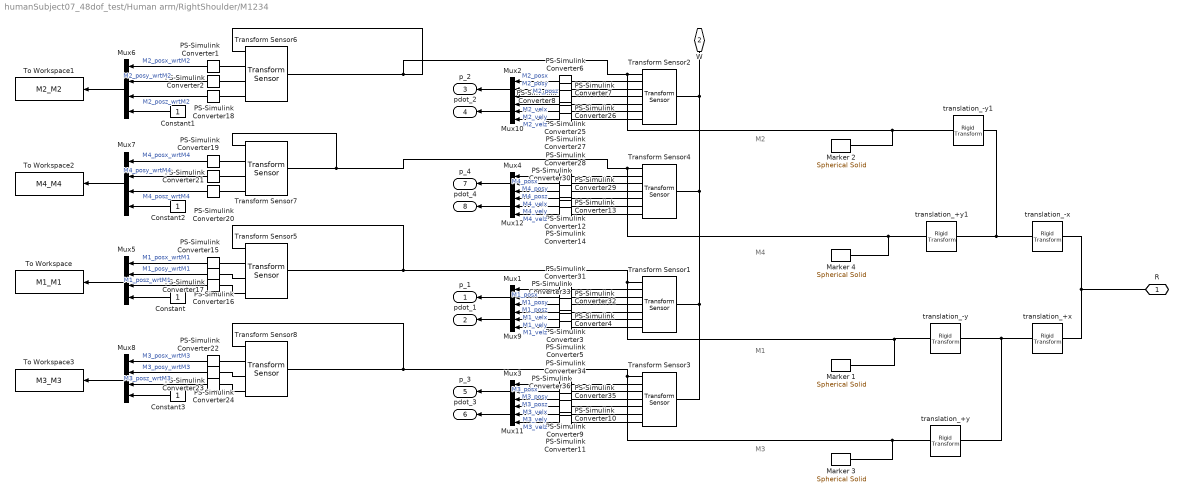
== system humanSubject07_48dof_test/Human arm/RightShoulder/M1234 ==
  note: M2
  note: M1
  note: M3
  note: M4
  Constant{,1..3} (4 alike) : Constant
  Marker {1..4} (4 alike) : sm_lib/Body Elements/Spherical Solid  GraphicAmbientColor=[0.15 0.15 0.15 1.0]  BasedOnType=Density  CenterOfMass=[0 0 0]  CenterOfMassUnits=m  GraphicDiffuseColor=[1.0 0.2 0.2]  Density=1000  DensityUnits=kg/m^3  DoExposeReferenceFrame=on  GraphicEmissiveColor=[0.0 0.0 0.0 1.0]  ExportEntireGeometry=off  SerializedExposedGeometries=<ExposedGeometries/>  SerializedFrames=<Frames/>  MarkerShape=Sphere  MarkerSize=10  GraphicType=FromGeometry  InertiaType=CalculateFromGeometry  Mass=1  MassUnits=kg  MomentsOfInertia=[1 1 1]  MomentsOfInertiaUnits=kg*m^2  GraphicOpacity=1.0  ProductsOfInertia=[0 0 0]  ProductsOfInertiaUnits=kg*m^2  GraphicShininess=75  GraphicSpecularColor=[0.5 0.5 0.5 1.0]  SphereRadius=arm.markers.radius  SphereRadiusUnits=m  GraphicVisPropType=SimpleVisualProperties
  Mux{1..4,9..12} (8 alike) : Mux  Inputs=3
  Mux{5..8} (4 alike) : Mux
  PS-Simulink Converter{1..36} (36 alike) : nesl_utility/PS-Simulink Converter  PhysicalDomain=network_engine_domain  SubClassName=ps_output  LeftPortType=input  RightPortType=output  PseudoPeriodic=off  Frequencies=[]  VectorFormat=inherit  Unit=inherit  AffineConversion=off
      settings: SourceProductBaseCode=SS,PW,VE
  To Workspace : ToWorkspace  VariableName=M1_M1  SaveFormat=Structure With Time  SampleTime=-1
  To Workspace1 : ToWorkspace  VariableName=M2_M2  SaveFormat=Structure With Time  SampleTime=-1
  To Workspace2 : ToWorkspace  VariableName=M4_M4  SaveFormat=Structure With Time  SampleTime=-1
  To Workspace3 : ToWorkspace  VariableName=M3_M3  SaveFormat=Structure With Time  SampleTime=-1
  Transform Sensor{1..4} (4 alike) : sm_lib/Frames and Transforms/Transform Sensor  MeasurementFrame=World  SenseAngle=off  SenseAxis=off  SenseAngle1=off  SenseAngle2=off  SenseAngle3=off  SenseQ=off  SenseR=off  SenseOmegaX=off  SenseOmegaY=off  SenseOmegaZ=off  SenseOmega1=off  SenseOmega2=off  SenseOmega3=off  SenseQDot=off  SenseRDot=off  SenseAlphaX=off  SenseAlphaY=off  SenseAlphaZ=off  SenseAlpha1=off  SenseAlpha2=off  SenseAlpha3=off  SenseQDDot=off  SenseRDDot=off  SenseX=on  SenseY=on  SenseZ=on  SenseRad=off  SenseAzim=off  SenseDist=off  SenseInc=off  SenseXDot=on  SenseYDot=on  SenseZDot=on  SenseRadDot=off  SenseAzimDot=off  SenseDistDot=off  SenseIncDot=off  SenseXDDot=off  SenseYDDot=off  SenseZDDot=off  SenseRadDDot=off  SenseAzimDDot=off  SenseDistDDot=off  SenseIncDDot=off
  Transform Sensor{5..8} (4 alike) : sm_lib/Frames and Transforms/Transform Sensor  MeasurementFrame=World  SenseAngle=off  SenseAxis=off  SenseAngle1=off  SenseAngle2=off  SenseAngle3=off  SenseQ=off  SenseR=off  SenseOmegaX=off  SenseOmegaY=off  SenseOmegaZ=off  SenseOmega1=off  SenseOmega2=off  SenseOmega3=off  SenseQDot=off  SenseRDot=off  SenseAlphaX=off  SenseAlphaY=off  SenseAlphaZ=off  SenseAlpha1=off  SenseAlpha2=off  SenseAlpha3=off  SenseQDDot=off  SenseRDDot=off  SenseX=on  SenseY=on  SenseZ=on  SenseRad=off  SenseAzim=off  SenseDist=off  SenseInc=off  SenseXDot=off  SenseYDot=off  SenseZDot=off  SenseRadDot=off  SenseAzimDot=off  SenseDistDot=off  SenseIncDot=off  SenseXDDot=off  SenseYDDot=off  SenseZDDot=off  SenseRadDDot=off  SenseAzimDDot=off  SenseDistDDot=off  SenseIncDDot=off
  translation_+x : sm_lib/Frames and Transforms/Rigid Transform  TranslationMethod=Cartesian  TranslationStandardOffset=0  TranslationLengthUnit=m  TranslationStandardAxis=+Z  TranslationCartesianOffset=[arm.shoulder.radius+arm.markers.radius 0 0]  TranslationROffset=0  TranslationROffsetUnits=m  TranslationZOffset=0  TranslationZOffsetUnits=m  TranslationThetaOffset=0  TranslationThetaOffsetUnits=deg  RotationMethod=None  RotationAngleUnits=rad  RotationStandardAxis=+Z  RotationAngle=pi/2  RotationArbitraryAxis=[1 0 0]  FollAlignAxisA=+X  BaseAlignAxisA=+Y  FollAlignAxisB=+Y  BaseAlignAxisB=+Z  RotationSequenceAxes=BaseAxes  RotationSequence=XYZ  RotationSequenceAngles=[pi/2, 0, 0]  RotationSequenceAnglesUnits=rad  RotationMatrix=[1 0 0; 0 1 0; 0 0 1]
  translation_+y : sm_lib/Frames and Transforms/Rigid Transform  TranslationMethod=Cartesian  TranslationStandardOffset=0  TranslationLengthUnit=m  TranslationStandardAxis=+Z  TranslationCartesianOffset=[0 arm.shoulder.length/4 0]  TranslationROffset=0  TranslationROffsetUnits=m  TranslationZOffset=0  TranslationZOffsetUnits=m  TranslationThetaOffset=0  TranslationThetaOffsetUnits=deg  RotationMethod=None  RotationAngleUnits=rad  RotationStandardAxis=+Z  RotationAngle=pi/2  RotationArbitraryAxis=[1 0 0]  FollAlignAxisA=+X  BaseAlignAxisA=+Y  FollAlignAxisB=+Y  BaseAlignAxisB=+Z  RotationSequenceAxes=BaseAxes  RotationSequence=XYZ  RotationSequenceAngles=[pi/2, 0, 0]  RotationSequenceAnglesUnits=rad  RotationMatrix=[1 0 0; 0 1 0; 0 0 1]
  translation_+y1 : sm_lib/Frames and Transforms/Rigid Transform  TranslationMethod=Cartesian  TranslationStandardOffset=0  TranslationLengthUnit=m  TranslationStandardAxis=+Z  TranslationCartesianOffset=[0 +arm.shoulder.length/4 0]  TranslationROffset=0  TranslationROffsetUnits=m  TranslationZOffset=0  TranslationZOffsetUnits=m  TranslationThetaOffset=0  TranslationThetaOffsetUnits=deg  RotationMethod=None  RotationAngleUnits=rad  RotationStandardAxis=+Z  RotationAngle=pi/2  RotationArbitraryAxis=[1 0 0]  FollAlignAxisA=+X  BaseAlignAxisA=+Y  FollAlignAxisB=+Y  BaseAlignAxisB=+Z  RotationSequenceAxes=BaseAxes  RotationSequence=XYZ  RotationSequenceAngles=[pi/2, 0, 0]  RotationSequenceAnglesUnits=rad  RotationMatrix=[1 0 0; 0 1 0; 0 0 1]
  translation_-x : sm_lib/Frames and Transforms/Rigid Transform  TranslationMethod=Cartesian  TranslationStandardOffset=0  TranslationLengthUnit=m  TranslationStandardAxis=+Z  TranslationCartesianOffset=[-arm.shoulder.radius-arm.markers.radius 0 0]  TranslationROffset=0  TranslationROffsetUnits=m  TranslationZOffset=0  TranslationZOffsetUnits=m  TranslationThetaOffset=0  TranslationThetaOffsetUnits=deg  RotationMethod=None  RotationAngleUnits=rad  RotationStandardAxis=+Z  RotationAngle=pi/2  RotationArbitraryAxis=[1 0 0]  FollAlignAxisA=+X  BaseAlignAxisA=+Y  FollAlignAxisB=+Y  BaseAlignAxisB=+Z  RotationSequenceAxes=BaseAxes  RotationSequence=XYZ  RotationSequenceAngles=[pi/2, 0, 0]  RotationSequenceAnglesUnits=rad  RotationMatrix=[1 0 0; 0 1 0; 0 0 1]
  translation_-y : sm_lib/Frames and Transforms/Rigid Transform  TranslationMethod=Cartesian  TranslationStandardOffset=0  TranslationLengthUnit=m  TranslationStandardAxis=+Z  TranslationCartesianOffset=[0 -arm.shoulder.length/4 0]  TranslationROffset=0  TranslationROffsetUnits=m  TranslationZOffset=0  TranslationZOffsetUnits=m  TranslationThetaOffset=0  TranslationThetaOffsetUnits=deg  RotationMethod=None  RotationAngleUnits=rad  RotationStandardAxis=+Z  RotationAngle=pi/2  RotationArbitraryAxis=[1 0 0]  FollAlignAxisA=+X  BaseAlignAxisA=+Y  FollAlignAxisB=+Y  BaseAlignAxisB=+Z  RotationSequenceAxes=BaseAxes  RotationSequence=XYZ  RotationSequenceAngles=[pi/2, 0, 0]  RotationSequenceAnglesUnits=rad  RotationMatrix=[1 0 0; 0 1 0; 0 0 1]
  translation_-y1 : sm_lib/Frames and Transforms/Rigid Transform  TranslationMethod=Cartesian  TranslationStandardOffset=0  TranslationLengthUnit=m  TranslationStandardAxis=+Z  TranslationCartesianOffset=[0 -arm.shoulder.length/4 0]  TranslationROffset=0  TranslationROffsetUnits=m  TranslationZOffset=0  TranslationZOffsetUnits=m  TranslationThetaOffset=0  TranslationThetaOffsetUnits=deg  RotationMethod=None  RotationAngleUnits=rad  RotationStandardAxis=+Z  RotationAngle=pi/2  RotationArbitraryAxis=[1 0 0]  FollAlignAxisA=+X  BaseAlignAxisA=+Y  FollAlignAxisB=+Y  BaseAlignAxisB=+Z  RotationSequenceAxes=BaseAxes  RotationSequence=XYZ  RotationSequenceAngles=[pi/2, 0, 0]  RotationSequenceAnglesUnits=rad  RotationMatrix=[1 0 0; 0 1 0; 0 0 1]
  R : PMIOPort  Side=Left
  W : PMIOPort  Port=2  Side=Left
  p_1 : Outport
  pdot_1 : Outport  Port=2
  p_2 : Outport  Port=3
  pdot_2 : Outport  Port=4
  p_3 : Outport  Port=5
  pdot_3 : Outport  Port=6
  p_4 : Outport  Port=7
  pdot_4 : Outport  Port=8
  wires:
  PS-Simulink Converter8/1 -> Mux2/3  "M2_posz"
  PS-Simulink Converter7/1 -> Mux2/2  "M2_posy"
  PS-Simulink Converter6/1 -> Mux2/1  "M2_posx"
  Mux5/1 -> To Workspace/1
  PS-Simulink Converter17/1 -> Mux5/3  "M1_posz_wrtM1"
  PS-Simulink Converter15/1 -> Mux5/1  "M1_posx_wrtM1"
  PS-Simulink Converter16/1 -> Mux5/2  "M1_posy_wrtM1"
  Constant/1 -> Mux5/4
  Mux6/1 -> To Workspace1/1
  PS-Simulink Converter1/1 -> Mux6/1  "M2_posx_wrtM2"
  PS-Simulink Converter2/1 -> Mux6/2  "M2_posy_wrtM2"
  Constant1/1 -> Mux6/4
  PS-Simulink Converter18/1 -> Mux6/3  "M2_posz_wrtM2"
  PS-Simulink Converter19/1 -> Mux7/1  "M4_posx_wrtM4"
  Constant2/1 -> Mux7/4
  PS-Simulink Converter21/1 -> Mux7/2  "M4_posy_wrtM4"
  Mux7/1 -> To Workspace2/1
  PS-Simulink Converter20/1 -> Mux7/3  "M4_posz_wrtM4"
  Constant3/1 -> Mux8/4
  PS-Simulink Converter22/1 -> Mux8/1  "M3_posx_wrtM3"
  PS-Simulink Converter24/1 -> Mux8/2  "M3_posy_wrtM3"
  Mux8/1 -> To Workspace3/1
  PS-Simulink Converter23/1 -> Mux8/3  "M3_posz_wrtM3"
  PS-Simulink Converter25/1 -> Mux10/1  "M2_velx"
  PS-Simulink Converter26/1 -> Mux10/2  "M2_vely"
  PS-Simulink Converter27/1 -> Mux10/3  "M2_velz"
  PS-Simulink Converter29/1 -> Mux4/2  "M4_posy"
  PS-Simulink Converter30/1 -> Mux4/3  "M4_posz"
  PS-Simulink Converter12/1 -> Mux12/1  "M4_velx"
  PS-Simulink Converter13/1 -> Mux12/2  "M4_vely"
  PS-Simulink Converter28/1 -> Mux4/1  "M4_posx"
  PS-Simulink Converter14/1 -> Mux12/3  "M4_velz"
  PS-Simulink Converter32/1 -> Mux1/2  "M1_posy"
  PS-Simulink Converter33/1 -> Mux1/3  "M1_posz"
  PS-Simulink Converter3/1 -> Mux9/1  "M1_velx"
  PS-Simulink Converter4/1 -> Mux9/2  "M1_vely"
  PS-Simulink Converter31/1 -> Mux1/1  "M1_posx"
  PS-Simulink Converter5/1 -> Mux9/3  "M1_velz"
  PS-Simulink Converter35/1 -> Mux3/2  "M3_posy"
  PS-Simulink Converter36/1 -> Mux3/3  "M3_posz"
  PS-Simulink Converter9/1 -> Mux11/1  "M3_velx"
  PS-Simulink Converter10/1 -> Mux11/2  "M3_vely"
  PS-Simulink Converter34/1 -> Mux3/1  "M3_posx"
  PS-Simulink Converter11/1 -> Mux11/3  "M3_velz"
  Mux1/1 -> p_1/1
  Mux9/1 -> pdot_1/1
  Mux10/1 -> pdot_2/1
  Mux2/1 -> p_2/1
  Mux11/1 -> pdot_3/1
  Mux3/1 -> p_3/1
  Mux12/1 -> pdot_4/1
  Mux4/1 -> p_4/1
  connections:
  translation_+x/LConn1 -- translation_-x/LConn1 -- R/RConn1
  translation_-y/LConn1 -- translation_+y/LConn1 -- translation_+x/RConn1
  translation_+y1/LConn1 -- translation_-y1/LConn1 -- translation_-x/RConn1
  Transform Sensor4/RConn1 -- translation_+y1/RConn1 -- Marker 4/RConn1 -- Transform Sensor7/LConn1 -- Transform Sensor7/RConn1
  Transform Sensor2/LConn1 -- W/RConn1 -- Transform Sensor3/LConn1 -- Transform Sensor1/LConn1 -- Transform Sensor4/LConn1
  PS-Simulink Converter7/LConn1 -- Transform Sensor2/RConn3
  Transform Sensor2/RConn4 -- PS-Simulink Converter8/LConn1
  PS-Simulink Converter6/LConn1 -- Transform Sensor2/RConn2
  PS-Simulink Converter17/LConn1 -- Transform Sensor5/RConn4
  Transform Sensor2/RConn1 -- translation_-y1/RConn1 -- Marker 2/RConn1 -- Transform Sensor6/RConn1 -- Transform Sensor6/LConn1
  PS-Simulink Converter1/LConn1 -- Transform Sensor6/RConn2
  PS-Simulink Converter18/LConn1 -- Transform Sensor6/RConn4
  PS-Simulink Converter2/LConn1 -- Transform Sensor6/RConn3
  PS-Simulink Converter20/LConn1 -- Transform Sensor7/RConn4
  PS-Simulink Converter21/LConn1 -- Transform Sensor7/RConn3
  PS-Simulink Converter19/LConn1 -- Transform Sensor7/RConn2
  PS-Simulink Converter24/LConn1 -- Transform Sensor8/RConn3
  PS-Simulink Converter23/LConn1 -- Transform Sensor8/RConn4
  PS-Simulink Converter22/LConn1 -- Transform Sensor8/RConn2
  Transform Sensor5/RConn2 -- PS-Simulink Converter15/LConn1
  Transform Sensor5/RConn3 -- PS-Simulink Converter16/LConn1
  Transform Sensor4/RConn4 -- PS-Simulink Converter30/LConn1
  PS-Simulink Converter29/LConn1 -- Transform Sensor4/RConn3
  PS-Simulink Converter28/LConn1 -- Transform Sensor4/RConn2
  Transform Sensor1/RConn1 -- Transform Sensor5/RConn1 -- Transform Sensor5/LConn1 -- Marker 1/RConn1 -- translation_-y/RConn1
  Transform Sensor1/RConn4 -- PS-Simulink Converter33/LConn1
  PS-Simulink Converter32/LConn1 -- Transform Sensor1/RConn3
  PS-Simulink Converter3/LConn1 -- Transform Sensor1/RConn5
  Transform Sensor1/RConn6 -- PS-Simulink Converter4/LConn1
  PS-Simulink Converter31/LConn1 -- Transform Sensor1/RConn2
  PS-Simulink Converter5/LConn1 -- Transform Sensor1/RConn7
  Transform Sensor3/RConn1 -- translation_+y/RConn1 -- Marker 3/RConn1 -- Transform Sensor8/RConn1 -- Transform Sensor8/LConn1
  Transform Sensor3/RConn4 -- PS-Simulink Converter36/LConn1
  PS-Simulink Converter35/LConn1 -- Transform Sensor3/RConn3
  PS-Simulink Converter34/LConn1 -- Transform Sensor3/RConn2
  PS-Simulink Converter9/LConn1 -- Transform Sensor3/RConn5
  PS-Simulink Converter10/LConn1 -- Transform Sensor3/RConn6
  PS-Simulink Converter11/LConn1 -- Transform Sensor3/RConn7
  PS-Simulink Converter12/LConn1 -- Transform Sensor4/RConn5
  PS-Simulink Converter13/LConn1 -- Transform Sensor4/RConn6
  PS-Simulink Converter14/LConn1 -- Transform Sensor4/RConn7
  PS-Simulink Converter25/LConn1 -- Transform Sensor2/RConn5
  PS-Simulink Converter26/LConn1 -- Transform Sensor2/RConn6
  PS-Simulink Converter27/LConn1 -- Transform Sensor2/RConn7

== system humanSubject07_48dof_test/Human arm/RightShoulder_joint/Sx_Sy ==
  jRightShoulder_rotx_AxisInvTransform : sm_lib/Frames and Transforms/Rigid Transform  TranslationMethod=Cartesian  TranslationStandardOffset=0  TranslationLengthUnit=m  TranslationStandardAxis=+Z  TranslationCartesianOffset=[0, 0, 0]  TranslationROffset=0  TranslationROffsetUnits=m  TranslationZOffset=0  TranslationZOffsetUnits=m  TranslationThetaOffset=0  TranslationThetaOffsetUnits=deg  RotationMethod=ArbitraryAxis  RotationAngleUnits=rad  RotationStandardAxis=+Z  RotationAngle=pi/2  RotationArbitraryAxis=[0, 1, 0]  FollAlignAxisA=+X  BaseAlignAxisA=+Y  FollAlignAxisB=+Y  BaseAlignAxisB=+Z  RotationSequenceAxes=FollowerAxes  RotationSequence=XYX  RotationSequenceAngles=[0 0 0]  RotationSequenceAnglesUnits=deg  RotationMatrix=[1 0 0; 0 1 0; 0 0 1]
  jRightShoulder_rotx_AxisInvTransform1 : sm_lib/Frames and Transforms/Rigid Transform  TranslationMethod=Cartesian  TranslationStandardOffset=0  TranslationLengthUnit=m  TranslationStandardAxis=+Z  TranslationCartesianOffset=[0, 0, 0]  TranslationROffset=0  TranslationROffsetUnits=m  TranslationZOffset=0  TranslationZOffsetUnits=m  TranslationThetaOffset=0  TranslationThetaOffsetUnits=deg  RotationMethod=ArbitraryAxis  RotationAngleUnits=rad  RotationStandardAxis=+Z  RotationAngle=pi/2  RotationArbitraryAxis=[0, 0, 1]  FollAlignAxisA=+X  BaseAlignAxisA=+Y  FollAlignAxisB=+Y  BaseAlignAxisB=+Z  RotationSequenceAxes=FollowerAxes  RotationSequence=XYX  RotationSequenceAngles=[0 0 0]  RotationSequenceAnglesUnits=deg  RotationMatrix=[1 0 0; 0 1 0; 0 0 1]
  Sx : PMIOPort  Side=Left
  Sy : PMIOPort  Port=2  Side=Right
  connections:
  Sx/RConn1 -- jRightShoulder_rotx_AxisInvTransform/LConn1
  jRightShoulder_rotx_AxisInvTransform/RConn1 -- jRightShoulder_rotx_AxisInvTransform1/LConn1
  jRightShoulder_rotx_AxisInvTransform1/RConn1 -- Sy/RConn1

== system humanSubject07_48dof_test/Human arm/RightShoulder_joint/Sy_Sz ==
  jRightShoulder_roty_AxisInvTransform : sm_lib/Frames and Transforms/Rigid Transform  TranslationMethod=Cartesian  TranslationStandardOffset=0  TranslationLengthUnit=m  TranslationStandardAxis=+Z  TranslationCartesianOffset=[0, 0, 0]  TranslationROffset=0  TranslationROffsetUnits=m  TranslationZOffset=0  TranslationZOffsetUnits=m  TranslationThetaOffset=0  TranslationThetaOffsetUnits=deg  RotationMethod=ArbitraryAxis  RotationAngleUnits=rad  RotationStandardAxis=+Z  RotationAngle=pi/2  RotationArbitraryAxis=[0, 1, 0]  FollAlignAxisA=+X  BaseAlignAxisA=+Y  FollAlignAxisB=+Y  BaseAlignAxisB=+Z  RotationSequenceAxes=FollowerAxes  RotationSequence=XYX  RotationSequenceAngles=[0 0 0]  RotationSequenceAnglesUnits=deg  RotationMatrix=[1 0 0; 0 1 0; 0 0 1]
  jRightShoulder_roty_AxisInvTransform1 : sm_lib/Frames and Transforms/Rigid Transform  TranslationMethod=Cartesian  TranslationStandardOffset=0  TranslationLengthUnit=m  TranslationStandardAxis=+Z  TranslationCartesianOffset=[0, 0, 0]  TranslationROffset=0  TranslationROffsetUnits=m  TranslationZOffset=0  TranslationZOffsetUnits=m  TranslationThetaOffset=0  TranslationThetaOffsetUnits=deg  RotationMethod=ArbitraryAxis  RotationAngleUnits=rad  RotationStandardAxis=+Z  RotationAngle=pi/2  RotationArbitraryAxis=[0, 0, 1]  FollAlignAxisA=+X  BaseAlignAxisA=+Y  FollAlignAxisB=+Y  BaseAlignAxisB=+Z  RotationSequenceAxes=FollowerAxes  RotationSequence=XYX  RotationSequenceAngles=[0 0 0]  RotationSequenceAnglesUnits=deg  RotationMatrix=[1 0 0; 0 1 0; 0 0 1]
  Sy : PMIOPort  Side=Left
  Sz : PMIOPort  Port=2  Side=Right
  connections:
  Sy/RConn1 -- jRightShoulder_roty_AxisInvTransform/LConn1
  jRightShoulder_roty_AxisInvTransform/RConn1 -- jRightShoulder_roty_AxisInvTransform1/LConn1
  jRightShoulder_roty_AxisInvTransform1/RConn1 -- Sz/RConn1

== system humanSubject07_48dof_test/Human arm/RightShoulder_joint/W_Sx ==
  jRightShoulder_rotx_OriginTransform : sm_lib/Frames and Transforms/Rigid Transform  TranslationMethod=Cartesian  TranslationStandardOffset=0  TranslationLengthUnit=m  TranslationStandardAxis=+Z  TranslationCartesianOffset=[0, 0, 0]  TranslationROffset=0  TranslationROffsetUnits=m  TranslationZOffset=0  TranslationZOffsetUnits=m  TranslationThetaOffset=0  TranslationThetaOffsetUnits=deg  RotationMethod=ArbitraryAxis  RotationAngleUnits=rad  RotationStandardAxis=+Z  RotationAngle=pi/2  RotationArbitraryAxis=[0 0 1]  FollAlignAxisA=+X  BaseAlignAxisA=+Y  FollAlignAxisB=+Y  BaseAlignAxisB=+Z  RotationSequenceAxes=BaseAxes  RotationSequence=XYZ  RotationSequenceAngles=[0, pi/2, 0]  RotationSequenceAnglesUnits=rad  RotationMatrix=[1 0 0; 0 1 0; 0 0 1]
  jRightShoulder_rotx_OriginTransform1 : sm_lib/Frames and Transforms/Rigid Transform  TranslationMethod=Cartesian  TranslationStandardOffset=0  TranslationLengthUnit=m  TranslationStandardAxis=+Z  TranslationCartesianOffset=[0, 0, 0]  TranslationROffset=0  TranslationROffsetUnits=m  TranslationZOffset=0  TranslationZOffsetUnits=m  TranslationThetaOffset=0  TranslationThetaOffsetUnits=deg  RotationMethod=ArbitraryAxis  RotationAngleUnits=rad  RotationStandardAxis=+Z  RotationAngle=pi/2  RotationArbitraryAxis=[1 0 0]  FollAlignAxisA=+X  BaseAlignAxisA=+Y  FollAlignAxisB=+Y  BaseAlignAxisB=+Z  RotationSequenceAxes=BaseAxes  RotationSequence=XYZ  RotationSequenceAngles=[0, pi/2, 0]  RotationSequenceAnglesUnits=rad  RotationMatrix=[1 0 0; 0 1 0; 0 0 1]
  W : PMIOPort  Side=Left
  Sx : PMIOPort  Port=2  Side=Right
  connections:
  W/RConn1 -- jRightShoulder_rotx_OriginTransform/LConn1
  jRightShoulder_rotx_OriginTransform1/LConn1 -- jRightShoulder_rotx_OriginTransform/RConn1
  jRightShoulder_rotx_OriginTransform1/RConn1 -- Sx/RConn1

== system humanSubject07_48dof_test/Human arm/Wrist_joint/F_elbow__Wx ==
  jRightShoulder_rotx_OriginTransform : sm_lib/Frames and Transforms/Rigid Transform  TranslationMethod=Cartesian  TranslationStandardOffset=0  TranslationLengthUnit=m  TranslationStandardAxis=+Z  TranslationCartesianOffset=[0, 0, 0]  TranslationROffset=0  TranslationROffsetUnits=m  TranslationZOffset=0  TranslationZOffsetUnits=m  TranslationThetaOffset=0  TranslationThetaOffsetUnits=deg  RotationMethod=ArbitraryAxis  RotationAngleUnits=rad  RotationStandardAxis=+Z  RotationAngle=pi/2  RotationArbitraryAxis=[0 0 1]  FollAlignAxisA=+X  BaseAlignAxisA=+Y  FollAlignAxisB=+Y  BaseAlignAxisB=+Z  RotationSequenceAxes=BaseAxes  RotationSequence=XYZ  RotationSequenceAngles=[0, pi/2, 0]  RotationSequenceAnglesUnits=rad  RotationMatrix=[1 0 0; 0 1 0; 0 0 1]
  jRightShoulder_rotx_OriginTransform1 : sm_lib/Frames and Transforms/Rigid Transform  TranslationMethod=Cartesian  TranslationStandardOffset=0  TranslationLengthUnit=m  TranslationStandardAxis=+Z  TranslationCartesianOffset=[0, 0, 0]  TranslationROffset=0  TranslationROffsetUnits=m  TranslationZOffset=0  TranslationZOffsetUnits=m  TranslationThetaOffset=0  TranslationThetaOffsetUnits=deg  RotationMethod=ArbitraryAxis  RotationAngleUnits=rad  RotationStandardAxis=+Z  RotationAngle=pi/2  RotationArbitraryAxis=[1 0 0]  FollAlignAxisA=+X  BaseAlignAxisA=+Y  FollAlignAxisB=+Y  BaseAlignAxisB=+Z  RotationSequenceAxes=BaseAxes  RotationSequence=XYZ  RotationSequenceAngles=[0, pi/2, 0]  RotationSequenceAnglesUnits=rad  RotationMatrix=[1 0 0; 0 1 0; 0 0 1]
  B_wrist : PMIOPort  Side=Left
  Wx : PMIOPort  Port=2  Side=Right
  connections:
  B_wrist/RConn1 -- jRightShoulder_rotx_OriginTransform/LConn1
  jRightShoulder_rotx_OriginTransform1/LConn1 -- jRightShoulder_rotx_OriginTransform/RConn1
  jRightShoulder_rotx_OriginTransform1/RConn1 -- Wx/RConn1

== system humanSubject07_48dof_test/Human arm/Wrist_joint/Wx_Wy ==
  jRightShoulder_rotx_AxisInvTransform2 : sm_lib/Frames and Transforms/Rigid Transform  TranslationMethod=Cartesian  TranslationStandardOffset=0  TranslationLengthUnit=m  TranslationStandardAxis=+Z  TranslationCartesianOffset=[0, 0, 0]  TranslationROffset=0  TranslationROffsetUnits=m  TranslationZOffset=0  TranslationZOffsetUnits=m  TranslationThetaOffset=0  TranslationThetaOffsetUnits=deg  RotationMethod=ArbitraryAxis  RotationAngleUnits=rad  RotationStandardAxis=+Z  RotationAngle=pi/2  RotationArbitraryAxis=[0, 1, 0]  FollAlignAxisA=+X  BaseAlignAxisA=+Y  FollAlignAxisB=+Y  BaseAlignAxisB=+Z  RotationSequenceAxes=FollowerAxes  RotationSequence=XYX  RotationSequenceAngles=[0 0 0]  RotationSequenceAnglesUnits=deg  RotationMatrix=[1 0 0; 0 1 0; 0 0 1]
  jRightShoulder_rotx_AxisInvTransform3 : sm_lib/Frames and Transforms/Rigid Transform  TranslationMethod=Cartesian  TranslationStandardOffset=0  TranslationLengthUnit=m  TranslationStandardAxis=+Z  TranslationCartesianOffset=[0, 0, 0]  TranslationROffset=0  TranslationROffsetUnits=m  TranslationZOffset=0  TranslationZOffsetUnits=m  TranslationThetaOffset=0  TranslationThetaOffsetUnits=deg  RotationMethod=ArbitraryAxis  RotationAngleUnits=rad  RotationStandardAxis=+Z  RotationAngle=pi/2  RotationArbitraryAxis=[0, 0, 1]  FollAlignAxisA=+X  BaseAlignAxisA=+Y  FollAlignAxisB=+Y  BaseAlignAxisB=+Z  RotationSequenceAxes=FollowerAxes  RotationSequence=XYX  RotationSequenceAngles=[0 0 0]  RotationSequenceAnglesUnits=deg  RotationMatrix=[1 0 0; 0 1 0; 0 0 1]
  Wx : PMIOPort  Side=Left
  Wy : PMIOPort  Port=2  Side=Right
  connections:
  jRightShoulder_rotx_AxisInvTransform3/RConn1 -- Wy/RConn1
  jRightShoulder_rotx_AxisInvTransform2/RConn1 -- jRightShoulder_rotx_AxisInvTransform3/LConn1
  Wx/RConn1 -- jRightShoulder_rotx_AxisInvTransform2/LConn1
